simulink model "Sim_rlc1"  (R2019a)
settings: Solver=VariableStepAuto  StartTime=0.0  StopTime=10.0  RelTol=1e-3
libraries: fl_lib x3, ee_lib x3, nesl_utility x1, powerlib x1
settings Model: Creator=zq001  LastModifiedBy=zq001
settings DebuggingCC: UnconnectedInputMsg=none  UnconnectedOutputMsg=none  UnconnectedLineMsg=none

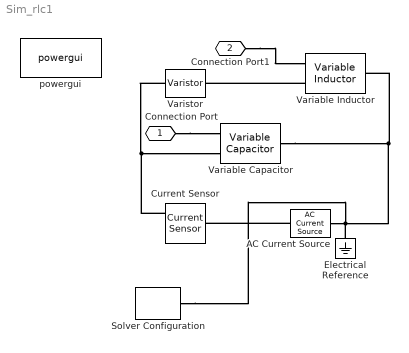
== system Sim_rlc1 ==
  AC Current Source : fl_lib/Electrical/Electrical Sources/AC Current Source  amp=1 A  shift=0 deg  frequency=60 Hz  omega=0 rad/s
      settings: SourceProductName=Simscape  SourceProductBaseCode=SS
  Current Sensor : fl_lib/Electrical/Electrical Sensors/Current Sensor
  Electrical Reference : fl_lib/Electrical/Electrical Elements/Electrical Reference
  Solver Configuration : nesl_utility/Solver Configuration  PhysicalDomain=network_engine_domain  SubClassName=solver  LeftPortType=input  RightPortType=generic  Tones=[]  Harmonics=[]  SimulateNoise=off  Profile=off  UseLocalSampling=off  EnableSwitchedLinearOptims=on  FrequencyDomain=off  UseCCode=off  RelTol=0.001  AbsTol=1e-06  MinStep=1e-09  ToWorkspace=off  RevertToSquareIcSolve=off  NumHomotopyIterations=100  PhasorMode=off  PhasorModeNumHarmonics=1  DoDC=off  ResidualTolerance=1e-09  UseLocalSolver=off  LocalSolverChoice=NE_BACKWARD_EULER_ADVANCER  LocalSolverSampleTime=0.001  DoFixedCost=off  MaxNonlinIter=3  MaxModeIter=2  LinearAlgebra=auto  EquationFormulation=NE_TIME_EF  DelaysMemoryBudget=1024  AutomaticFiltering=on  FilteringTimeConstant=0.001  PartitionStorageMethod=AS_NEEDED  PartitionMemoryBudget=1024  PartitionMethod=ROBUST
  Variable Capacitor : ee_lib/Passive/Variable Capacitor  prm=2  Cmin=1e-9 F  r=1e-6 Ohm  v0=0 V  q0=0 C
      settings: SourceProductName=Simscape Electrical  SourceProductBaseCode=PS
  Variable Inductor : ee_lib/Passive/Variable Inductor  prm=1  Lmin=1e-6 H  g=1e-9 1/Ohm  i0=0 A  phi0=0 Wb
      settings: SourceProductName=Simscape Electrical  SourceProductBaseCode=PS
  Varistor : ee_lib/Passive/Varistor  prm=1  vclamp=260 V  roff=3e8 Ohm  ron=1 Ohm  vln=130 V  vnu=300 V  rLeak=3e8 Ohm  alphaNormal=45  rUpturn=0.07 Ohm  rseries=100e-6 Ohm  c=4.4 nF  v_varistor_specify=off  v_varistor_priority=None  v_varistor=0 V  v_varistor_nominal_specify=off  v_varistor_nominal_unit=V  v_varistor_nominal_value=1
      settings: SourceProductName=Simscape Electrical  SourceProductBaseCode=PS
  powergui : powerlib/powergui  Priority=1  SimulationMode=Continuous  SampleTime=50e-6  frequency=60  Iterations=50  frequencyindice=60  Pbase=100e6  ErrMax=1e-4  UnitsV=kV  UnitsW=MW  buscounter=0  FunctionMessages=off  echomessages=off  EnableUseOfTLC=off  CurrentSourceSwitches=off  DisableSnubberDevices=off  DisableRonSwitches=off  DisableVfSwitches=off  DisplayEquations=off  AutomaticDiscreteSolvers=off  SolverType=Tustin/Backward Euler (TBE)  Interpol=off  ExternalGateDelay=off  methode=off  Ts=100  x0status=blocks  SPID=on  SwTol=0  HookPort=off  NonlinearTolerance=0  nMaxIteration=15  ContinueOnMaxIteration=off  RestoreLinks=warning  ResistiveCurrentMeasurement=off  Frange=[0:2:500]  Ylog=off  Xlog=on  ShowGrid=off  save=off  variable=ZData  structure=0  ZoomFFT=off  StartTime=0.0  cycles=1  DisplayStyle=1  fundamental=60  FreqAxis=off  MaxFrequency=1000  frequencyindicesteady=1  RmsSteady=1  display=off
      settings: SourceProductName=Simscape Electrical
  Connection Port : PMIOPort  Side=Left
  Connection Port1 : PMIOPort  Port=2  Side=Left
  connections:
  Varistor/LConn1 -- Current Sensor/RConn2 -- Variable Capacitor/LConn2
  Variable Inductor/LConn2 -- Varistor/RConn1
  Variable Capacitor/RConn1 -- Electrical Reference/LConn1 -- Solver Configuration/RConn1 -- AC Current Source/RConn1 -- Variable Inductor/RConn1
  AC Current Source/LConn1 -- Current Sensor/LConn1
  Connection Port/RConn1 -- Variable Capacitor/LConn1
  Connection Port1/RConn1 -- Variable Inductor/LConn1
